simulink model "lab-week-9"  (R2018a)
settings: Solver=FixedStepAuto  StartTime=0.0  StopTime=400  FixedStep=0.1  RelTol=1e-3
undefined symbols (not defined in the file): serial
libraries: instrumentlib x4, dspstat3 x1, simulink x1, sldrtlib x1
settings Model: SimulationMode=accelerator  Creator=gwilfong  LastModifiedBy=katherto
settings CodeAppCC: StateflowObjectComments=on

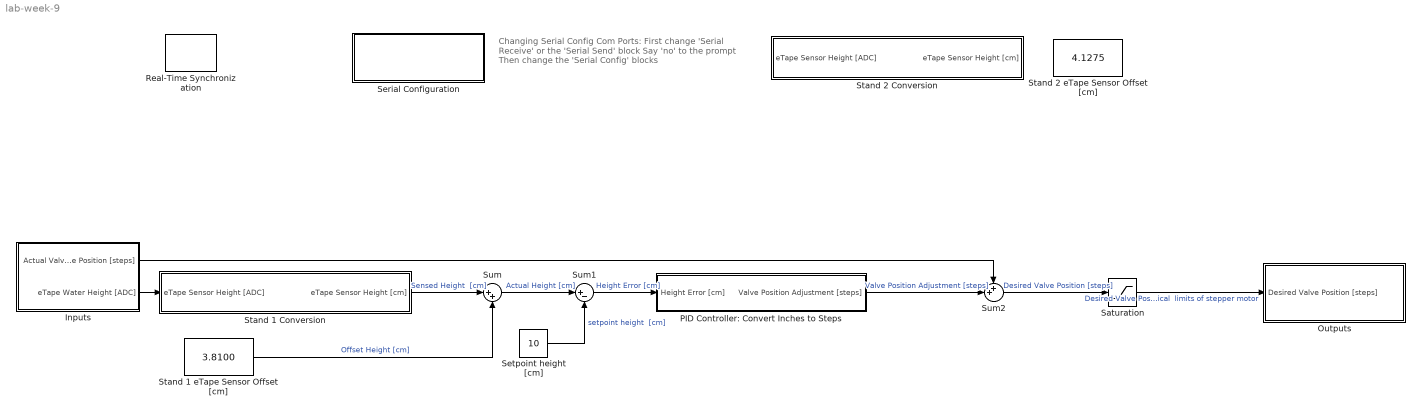
== system lab-week-9 ==
  note: Changing Serial Config Com Ports:
      | First change 'Serial Receive' or the 'Serial Send' block
      | Say 'no' to the prompt
      | Then change the 'Serial Config' blocks
  Inputs : Subsystem
  Outputs : Subsystem
  PID Controller: Convert Inches to Steps : Subsystem
  Real-Time Synchronization : sldrtlib/Real-Time Synchronization  SampleTime=0.1  MaxMissedTicks=10  ShowMissedTicks=off  YieldWhenWaiting=off
  Saturation : Saturate  UpperLimit=1020  LowerLimit=0
  Serial Configuration : Subsystem
  Setpoint height [cm] : Constant  Value=10
  Stand 1 Conversion : Subsystem
  Stand 1 eTape Sensor Offset [cm] : Constant  Value=3.8100
  Stand 2 Conversion : Subsystem
  Stand 2 eTape Sensor Offset [cm] : Constant  Value=4.1275
  Sum : Sum  Inputs=|++
  Sum1 : Sum  Inputs=|+-
  Sum2 : Sum  Inputs=++|
  wires:
  Inputs/2(eTape Water Height [ADC]) -> Stand 1 Conversion/1(eTape Sensor Height [ADC])
  Stand 1 Conversion/1(eTape Sensor Height [cm]) -> Sum/1  "Sensed Height  [cm]"
  Stand 1 eTape Sensor Offset [cm]/1 -> Sum/2  "Offset Height [cm]"
  Sum/1 -> Sum1/1  "Actual Height [cm]"
  Setpoint height [cm]/1 -> Sum1/2  "setpoint height  [cm]"
  Sum1/1 -> PID Controller: Convert Inches to Steps/1(Height Error [cm])  "Height Error [cm]"
  PID Controller: Convert Inches to Steps/1(Valve Position Adjustment [steps]) -> Sum2/2  "Valve Position Adjustment [steps]"
  Inputs/1(Actual Valve Position [steps]) -> Sum2/1
  Sum2/1 -> Saturation/1  "Desired Valve Position [steps]"
  Saturation/1 -> Outputs/1(Desired Valve Position [steps])  "Desired Valve Position  [steps] limited by physical  limits of stepper motor"

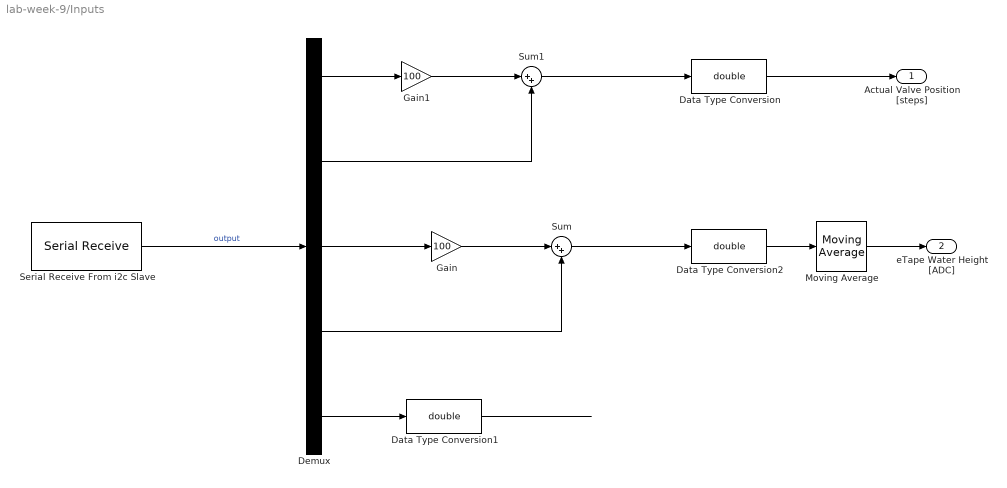
== system lab-week-9/Inputs ==
  Data Type Conversion : DataTypeConversion  OutDataTypeStr=double
  Data Type Conversion1 : DataTypeConversion  OutDataTypeStr=double
  Data Type Conversion2 : DataTypeConversion  OutDataTypeStr=double
  Demux : Demux  Outputs=5
  Gain : Gain  Gain=100
  Gain1 : Gain  Gain=100
  Moving Average : dspstat3/Moving Average  Method=Sliding window  ForgettingFactorPort=off  SpecifyWindowLength=on  WindowLength=10  ForgettingFactor=0.9  SimulateUsing=Code generation
  Serial Receive From i2c Slave : instrumentlib/Serial Receive  ComPortMenu=<Please select a port...>  ComPort=COM5  ObjConstructor=serial('COM5');  Terminator=<none>  DataSize="[5  1]"  DataType=uint8  EnableBlockingMode=on  ActionDataUnavailable=Output last received value  CustomValue=0  SampleTime=.1
  Sum : Sum  Inputs=|++
  Sum1 : Sum  Inputs=|++
  Actual Valve Position [steps] : Outport
  eTape Water Height [ADC] : Outport  Port=2
  wires:
  Serial Receive From i2c Slave/1 -> Demux/1  "output"
  Gain/1 -> Sum/1
  Data Type Conversion/1 -> Actual Valve Position [steps]/1
  Gain1/1 -> Sum1/1
  Demux/3 -> Gain/1
  Demux/4 -> Sum/2
  Demux/1 -> Gain1/1
  Demux/2 -> Sum1/2
  Sum1/1 -> Data Type Conversion/1
  Data Type Conversion2/1 -> Moving Average/1
  Sum/1 -> Data Type Conversion2/1
  Demux/5 -> Data Type Conversion1/1
  Data Type Conversion1/1 -> ?
  Moving Average/1 -> eTape Water Height [ADC]/1

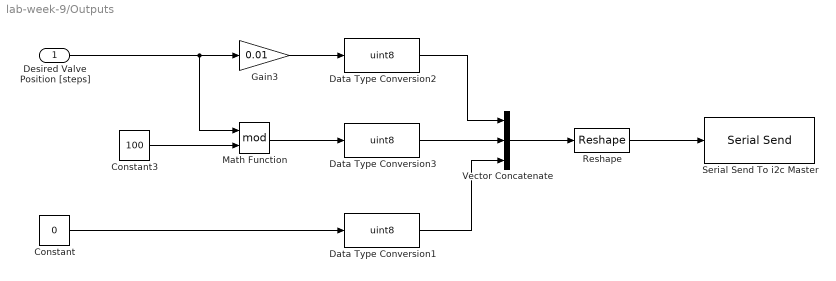
== system lab-week-9/Outputs ==
  Desired Valve Position [steps] : Inport
  Constant : Constant  Value=0
  Constant3 : Constant  Value=100
  Data Type Conversion1 : DataTypeConversion  OutDataTypeStr=uint8
  Data Type Conversion2 : DataTypeConversion  OutDataTypeStr=uint8
  Data Type Conversion3 : DataTypeConversion  OutDataTypeStr=uint8
  Gain3 : Gain  Gain=0.01
  Math Function : Math  Operator=mod  SaturateOnIntegerOverflow=on
  Reshape : Reshape  OutputDimensionality=Customize  OutputDimensions=[3,1]
  Serial Send To i2c Master : instrumentlib/Serial Send  ComPortMenu=<Please select a port...>  ComPort=COM4  ObjConstructor=serial('COM4');  Terminator=<none>  EnableBlockingMode=on
  Vector Concatenate : Concatenate  NumInputs=3
  wires:
  Constant/1 -> Data Type Conversion1/1
  Constant3/1 -> Math Function/2
  Gain3/1 -> Data Type Conversion2/1
  Math Function/1 -> Data Type Conversion3/1
  Vector Concatenate/1 -> Reshape/1
  Reshape/1 -> Serial Send To i2c Master/1
  Data Type Conversion2/1 -> Vector Concatenate/1
  Data Type Conversion3/1 -> Vector Concatenate/2
  Desired Valve Position [steps]/1 -> Math Function/1, Gain3/1
  Data Type Conversion1/1 -> Vector Concatenate/3

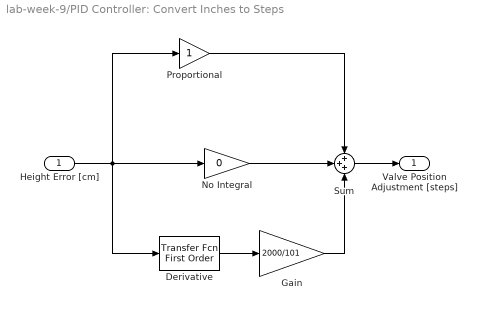
== system lab-week-9/PID Controller: Convert Inches to Steps ==
  Height Error [cm] : Inport
  Derivative : simulink/Discrete/Transfer Fcn First Order  PoleZ=-100  ICPrevOutput=0.0  DoSatur=off
      settings: SourceProductName=Simulink
  Gain : Gain  Gain=2000/101
  No Integral : Gain  Gain=0
  Proportional : Gain
  Sum : Sum  Inputs=+++
  Valve Position Adjustment [steps] : Outport
  wires:
  Sum/1 -> Valve Position Adjustment [steps]/1
  Height Error [cm]/1 -> Derivative/1, No Integral/1, Proportional/1
  Proportional/1 -> Sum/1
  No Integral/1 -> Sum/2
  Derivative/1 -> Gain/1
  Gain/1 -> Sum/3

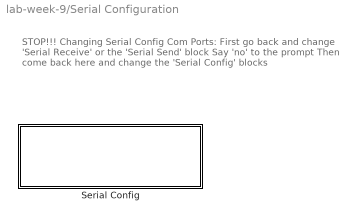
== system lab-week-9/Serial Configuration ==
  note: STOP!!!
      | Changing Serial Config Com Ports:
      | First go back and change 'Serial Receive' or the 'Serial Send' block
      | Say 'no' to the prompt
      | Then come back here and change the 'Serial Config' blocks
  Serial Config : Subsystem

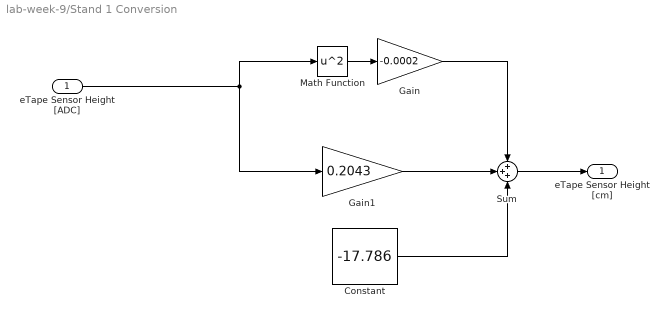
== system lab-week-9/Stand 1 Conversion ==
  eTape Sensor Height [ADC] : Inport
  Constant : Constant  Value=-17.786
  Gain : Gain  Gain=-0.0002
  Gain1 : Gain  Gain=0.2043
  Math Function : Math  Operator=square  SaturateOnIntegerOverflow=on
  Sum : Sum  Inputs=+++
  eTape Sensor Height [cm] : Outport
  wires:
  Constant/1 -> Sum/3
  Gain1/1 -> Sum/2
  eTape Sensor Height [ADC]/1 -> Math Function/1, Gain1/1
  Sum/1 -> eTape Sensor Height [cm]/1
  Math Function/1 -> Gain/1
  Gain/1 -> Sum/1

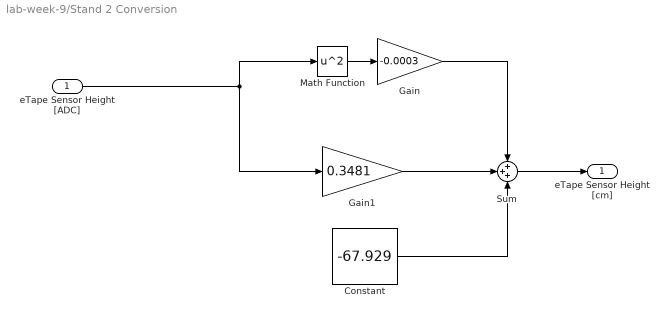
== system lab-week-9/Stand 2 Conversion ==
  eTape Sensor Height [ADC] : Inport
  Constant : Constant  Value=-67.929
  Gain : Gain  Gain=-0.0003
  Gain1 : Gain  Gain=0.3481
  Math Function : Math  Operator=square  SaturateOnIntegerOverflow=on
  Sum : Sum  Inputs=+++
  eTape Sensor Height [cm] : Outport
  wires:
  Constant/1 -> Sum/3
  Gain1/1 -> Sum/2
  eTape Sensor Height [ADC]/1 -> Math Function/1, Gain1/1
  Sum/1 -> eTape Sensor Height [cm]/1
  Math Function/1 -> Gain/1
  Gain/1 -> Sum/1

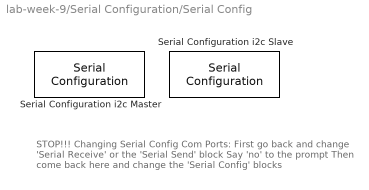
== system lab-week-9/Serial Configuration/Serial Config ==
  note: STOP!!!
      | Changing Serial Config Com Ports:
      | First go back and change 'Serial Receive' or the 'Serial Send' block
      | Say 'no' to the prompt
      | Then come back here and change the 'Serial Config' blocks
  Serial Configuration i2c Master : instrumentlib/Serial Configuration  Priority=-200000  ComPortMenu=COM4  ComPort=COM4  ObjConstructor=serial('COM4');  BaudRate=9600  DataBits=8  Parity=none  StopBits=1  FlowControl=none  Timeout=10  ByteOrder=LittleEndian
  Serial Configuration i2c Slave : instrumentlib/Serial Configuration  Priority=-200000  ComPortMenu=COM5  ComPort=COM5  ObjConstructor=serial('COM5');  BaudRate=9600  DataBits=8  Parity=none  StopBits=1  FlowControl=none  Timeout=10  ByteOrder=LittleEndian
